simulink model "design"  (R2020a)
settings: Solver=VariableStepAuto  StartTime=0.0  StopTime=10.0  RelTol=1e-3
undefined symbols (not defined in the file): A, B, N
libraries: lib x1
settings Model: Creator=sreeram  LastModifiedBy=sreeram

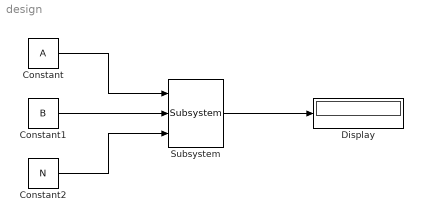
== system design ==
  Constant : Constant  Value=A
  Constant1 : Constant  Value=B
  Constant2 : Constant  Value=N
  Display : Display
  Subsystem : lib/Subsystem  A=0  B=0  N=0
  wires:
  Constant/1 -> Subsystem/1
  Constant1/1 -> Subsystem/2
  Constant2/1 -> Subsystem/3
  Subsystem/1 -> Display/1
